simulink model "simulation_commande_lineaire"  (R2020a)
settings: Solver=ode23  StartTime=0.0  StopTime=100  RelTol=1e-6
values from neighbouring files (symbols this model uses):
  A = [0 1;0 0]    [Adaptive_Control.m]    (also in Adaptive_Control_Linear.m = [0 1;a1 a2]; HGO.m = [0 1;-1 -1]; Non_linear_observers_.m; feedback-integrator.m = [1 1;0 0])
  a = 1    [Adap.m]    (also in Adaptive_control_Non_linear.m = 2; HOSM.m; projet_AAV.m; sys.m)
  B = [0;1]    [Adaptive_Control.m]    (also in Adaptive_Control_Linear.m = [0;b]; Non_linear_observers_.m; feedback-integrator.m = [0;1+b]; mini_projet.m = [0;1+b])
  b = 2    [Adaptive_Control_Linear.m]    (also in Adaptive_control_Non_linear.m; HOSM.m = 1; feedback-integrator.m = 3; mini_projet.m = 3)
  K = [Kaug(1),Kaug(2)]    [Adaptive_Control_Linear.m]    (also in projet_AAV.m = place(A, B, [-1,-2]))
settings Model: Creator=lenovo  LastModifiedBy=lenovo
settings SolverCC: AlgebraicLoopSolver=LineSearch

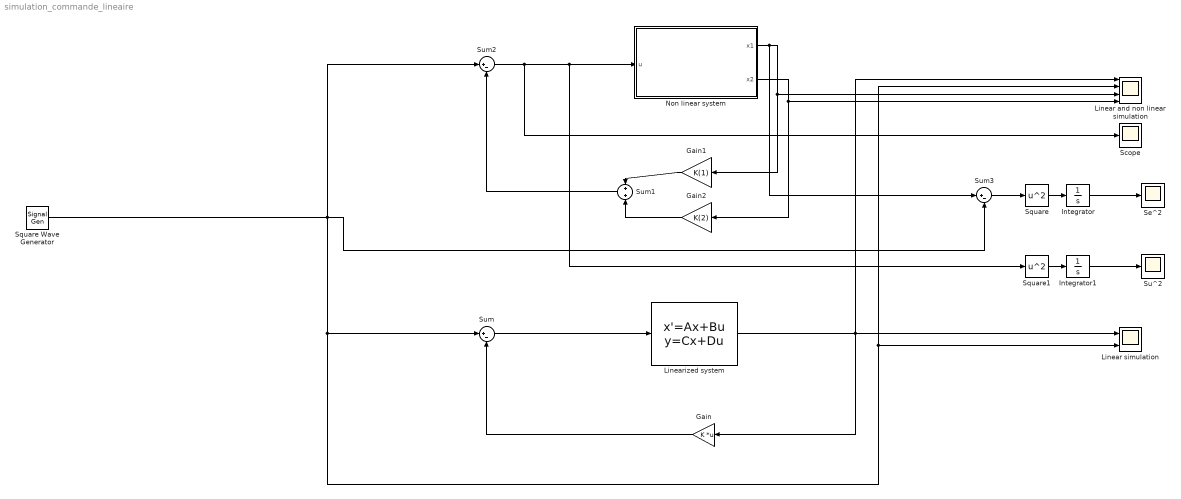
== system simulation_commande_lineaire ==
  Gain : Gain  Gain=K  Multiplication=Matrix(K*u)
  Gain1 : Gain  Gain=K(1)
  Gain2 : Gain  Gain=K(2)
  Integrator : Integrator
  Integrator1 : Integrator
  Linear and non linear simulation : Scope  NumInputPorts=4
  Linear simulation : Scope  NumInputPorts=2
  Linearized system : StateSpace  A=A  B=B  C=[1 0;0 1]  D=[0;0]  InitialCondition=2
  Non linear system : Subsystem
  Scope : Scope
  Se^2 : Scope
  Square : Math  Operator=square  SaturateOnIntegerOverflow=on
  Square Wave Generator : SignalGenerator  WaveForm=square  Frequency=0.1  Units=rad/sec
  Square1 : Math  Operator=square  SaturateOnIntegerOverflow=on
  Su^2 : Scope
  Sum : Sum  Inputs=|+-
  Sum1 : Sum  Inputs=+|+
  Sum2 : Sum  Inputs=|+-
  Sum3 : Sum  Inputs=|+-
  wires:
  Linearized system/1 -> Linear and non linear simulation/1, Linear simulation/1, Gain/1
  Sum/1 -> Linearized system/1
  Square Wave Generator/1 -> Sum3/2, Sum2/1, Sum/1, Linear and non linear simulation/2, Linear simulation/2
  Gain/1 -> Sum/2
  Non linear system/1(x1) -> Sum3/1, Gain1/1, Linear and non linear simulation/3
  Non linear system/2(x2) -> Gain2/1, Linear and non linear simulation/4
  Gain2/1 -> Sum1/2
  Gain1/1 -> Sum1/1
  Sum1/1 -> Sum2/2
  Square/1 -> Integrator/1
  Sum3/1 -> Square/1
  Integrator/1 -> Se^2/1
  Integrator1/1 -> Su^2/1
  Square1/1 -> Integrator1/1
  Sum2/1 -> Scope/1, Square1/1, Non linear system/1(u)

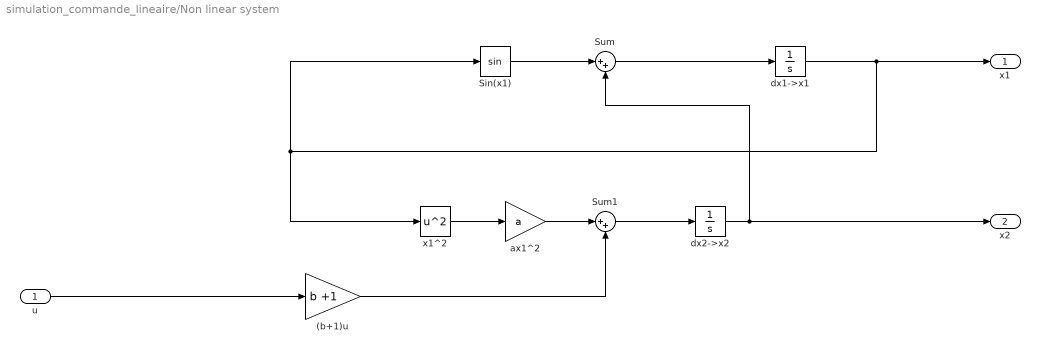
== system simulation_commande_lineaire/Non linear system ==
  u : Inport
  (b+1)u : Gain  Gain=b +1
  Sin(x1) : Trigonometry
  Sum : Sum  Inputs=|++
  Sum1 : Sum  Inputs=|++
  ax1^2 : Gain  Gain=a
  dx1->x1 : Integrator
  dx2->x2 : Integrator
  x1^2 : Math  Operator=square  SaturateOnIntegerOverflow=on
  x1 : Outport
  x2 : Outport  Port=2
  wires:
  (b+1)u/1 -> Sum1/2
  dx2->x2/1 -> x2/1, Sum/2
  u/1 -> (b+1)u/1
  ax1^2/1 -> Sum1/1
  dx1->x1/1 -> Sin(x1)/1, x1^2/1, x1/1
  Sin(x1)/1 -> Sum/1
  x1^2/1 -> ax1^2/1
  Sum1/1 -> dx2->x2/1
  Sum/1 -> dx1->x1/1
